simulink model "Assignment2FAST"  (R2022a)
settings: Solver=FixedStepAuto  StartTime=0.0  StopTime=inf  FixedStep=0.01  RelTol=1e-3
values from neighbouring files (symbols this model uses):
  WaypointList = [ 5,  0, pi/2 ... (first row only)    [A1_ScriptForWPMatrix.m]    (also in WList.mat = [5 5 -5 -5 0 3 -3 0 3 0 0 5 ... (30 elements, 10x3)])
undefined symbols (not defined in the file or in its folder): Angular, Linear
libraries: robotlib x3
settings Model: Creator=jacopo  LastModifiedBy=jacopo
settings OptimizationCC: EnhancedBackFolding=on  PassReuseOutputArgsAs=Individual arguments  ZeroExternalMemoryAtStartup=off  ZeroInternalMemoryAtStartup=off  MaxStackSize=64  OptimizeBlockOrder=speed  DifferentSizesBufferReuse=on  OptimizationCustomize=off  EfficientTunableParamExpr=on
settings DebuggingCC: ParameterTunabilityLossMsg=error
settings HardwareCC: ProdBitPerPointer=32  ProdBitPerSizeT=32  ProdBitPerPtrDiffT=32  ProdLargestAtomicFloat=None  ProdIntDivRoundTo=Undefined  ProdEndianess=Unspecified  ProdWordSize=32  ProdHWDeviceType=Generic->Unspecified (assume 32-bit Generic)
settings SFSimCC: MATLABDynamicMemAlloc=off
settings RTWCC: SystemTargetFile=ert.tlc  HardwareBoard=Robot Operating System (ROS)  TLCOptions="-aInlineSetEventsForThisBaseRateFcn=TLC_FALSE -aSuppressMultiTaskScheduler=TLC_FALSE  -aRateBasedStepFcn=0"  TemplateMakefile=ert_default_tmf  Toolchain=Catkin  TargetLang=C++
settings CodeAppCC: ForceParamTrailComments=on  IgnoreCustomStorageClasses=off  OperatorAnnotations=on  SimulinkDataObjDesc=on  SFDataObjDesc=on  InsertBlockDesc=on

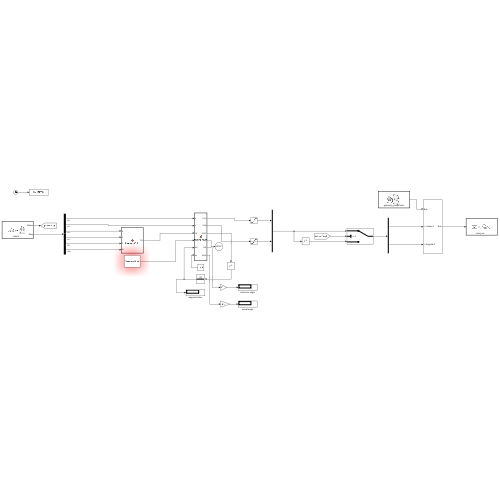
[thumbnail: Simulink's stored preview of the top-level diagram]
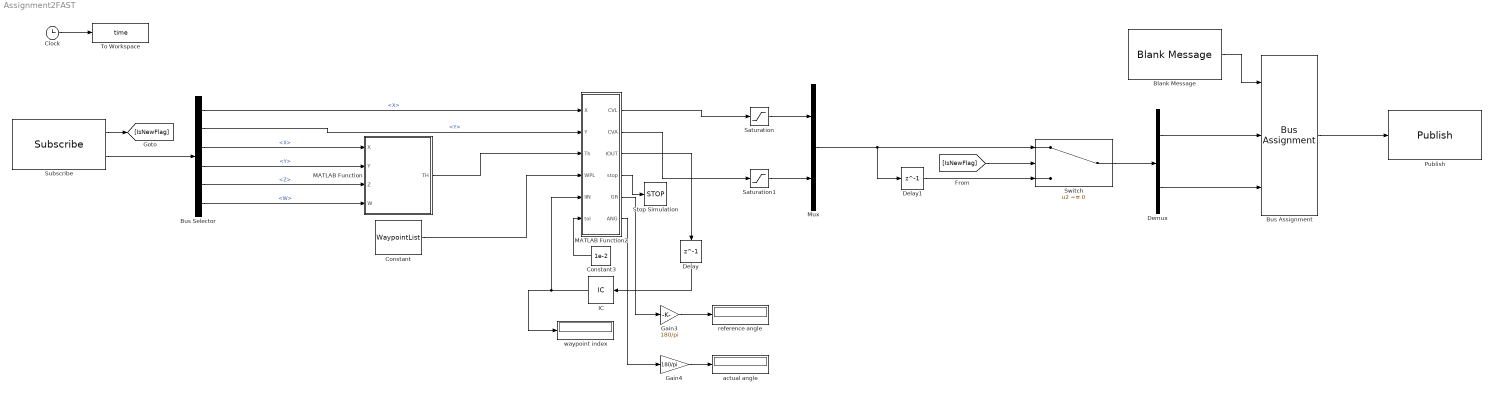
== system Assignment2FAST ==
  Blank Message : robotlib/Blank Message  messageClass=Message  entityType=geometry_msgs/Twist  messageType=geometry_msgs/Twist  SampleTime=inf  legacyBusStruct=off
  Bus Assignment : BusAssignment  AssignedSignals=Linear.X,Angular.Z
  Bus Selector : BusSelector  OutputSignals=Pose.Pose.Position.X,Pose.Pose.Position.Y,Pose.Pose.Orientation.X,Pose.Pose.Orientation.Y,Pose.Pose.Orientation.Z,Pose.Pose.Orientation.W
  Clock : Clock
  Constant : Constant  Value=WaypointList
  Constant3 : Constant  Value=1e-2
  Delay : Delay  DelayLength=1
  Delay1 : Delay  DelayLength=1
  Demux : Demux  Outputs=2
  Gain3 : Gain  Gain=180/pi
  Gain4 : Gain  Gain=180/pi
  IC : InitialCondition
  MATLAB Function : MATLAB Function  TreatAsAtomicUnit=on
  MATLAB Function2 : MATLAB Function  TreatAsAtomicUnit=on
  Mux : Mux  Inputs=2
  Publish : robotlib/Publish  topicSource=Select from ROS network  topic=/cmd_vel  messageType=geometry_msgs/Twist  legacyBusStruct=off  messageQueueLength=1
  Saturation : Saturate  UpperLimit=0.2  LowerLimit=-0.2
  Saturation1 : Saturate  UpperLimit=0.4  LowerLimit=-0.4
  Stop Simulation : Stop
  Subscribe : robotlib/Subscribe  topicSource=Select from ROS network  topic=/odom  messageType=nav_msgs/Odometry  SampleTime=-1  legacyBusStruct=off  messageQueueLength=1
  Switch : Switch  Criteria=u2 ~= 0  SaturateOnIntegerOverflow=off  InputSameDT=off
  To Workspace : ToWorkspace  VariableName=time  SampleTime=-1
  actual angle : Display
  reference angle : Display
  waypoint index : Display
  wires:
  Subscribe/2 -> Bus Selector/1
  Bus Selector/3 -> MATLAB Function/1(X)  "<X>"
  Bus Selector/4 -> MATLAB Function/2(Y)  "<Y>"
  Bus Selector/5 -> MATLAB Function/3(Z)  "<Z>"
  Bus Selector/6 -> MATLAB Function/4(W)  "<W>"
  Constant/1 -> MATLAB Function2/4(WPL)
  MATLAB Function/1(TH) -> MATLAB Function2/3(Th)
  Bus Selector/2 -> MATLAB Function2/2(Y)  "<Y>"
  Bus Selector/1 -> MATLAB Function2/1(X)  "<X>"
  MATLAB Function2/1(CVL) -> Saturation/1
  MATLAB Function2/2(CVA) -> Saturation1/1
  Subscribe/1 -> [IsNewFlag]
  [IsNewFlag] -> Switch/2
  Saturation/1 -> Mux/1
  Saturation1/1 -> Mux/2
  Mux/1 -> Delay1/1, Switch/1
  Switch/1 -> Demux/1
  Blank Message/1 -> Bus Assignment/1
  Demux/1 -> Bus Assignment/2
  Demux/2 -> Bus Assignment/3
  Bus Assignment/1 -> Publish/1
  Clock/1 -> To Workspace/1
  IC/1 -> waypoint index/1, MATLAB Function2/5(IIN)
  Delay/1 -> IC/1
  MATLAB Function2/3(IOUT) -> Delay/1
  MATLAB Function2/4(stop) -> Stop Simulation/1
  Delay1/1 -> Switch/3
  Constant3/1 -> MATLAB Function2/6(tol)
  MATLAB Function2/5(GR) -> Gain3/1
  Gain3/1 -> reference angle/1
  Gain4/1 -> actual angle/1
  MATLAB Function2/6(ANG) -> Gain4/1

== matlab function Assignment2FAST/MATLAB Function ==
  data: X input; TH output; Y input; Z input; W input
function TH = fromQuat2Eu(X, Y, Z, W)

ANGLE = quat2eul([W, X, Y, Z]);

TH = ANGLE(1);

== matlab function Assignment2FAST/MATLAB Function2 ==
  data: X input; CVL output; Y input; Th input; WPL input; CVA output; IOUT output; IIN input; stop output; tol input; GR output; ANG output
function [CVL, CVA, IOUT, stop, GR, ANG] = FBRegulator(X, Y, Th, WPL, IIN, tol)

kPL = 1;
kPA = 1.4;

POSr = WPL(IIN, :);

Xr = POSr(1); Yr = POSr(2); Thr = POSr(3);

Z = (Xr - X) + 1i*(Yr - Y);

dist = abs(Z);

Gr = angle(Z);

if (Th > tol) && (- pi + tol < Gr && Gr < - pi/2 - tol)
    Gr = Gr + 2*pi;
elseif (- pi + tol < Th && Th < - pi/2 - tol) && (Gr > tol)
    Th = Th + 2*pi;
end


errTh = Gr - Th;
GR = Gr;

ANG = Th;

CVL = kPL*0.2;
CVA = kPA*errTh;


if dist <= 0.05 
   stop = 0;
   IOUT = IIN + 1;
   if IIN == 10
       CVL = 0;
       CVA = 0;
       stop = 1;
   end
else
    IOUT = IIN;
    stop = 0;
end
